simulink model "accBasedController_Simulation"  (R2020a)
settings: Solver=VariableStepAuto  StartTime=0  StopTime=20  FixedStep=0.001  RelTol=1e-3
values from neighbouring files (symbols this model uses):
  A = [0 0 0 1 0 0;      0 0 0 0 1 0;      0 0 0 0 0 1;      -Ka/Jh Ka/Jh 0 0 0 0;     Ka/Je -(Ks + Ka)/Je Ks/Je 0 0 0;      0 Ks/Ja -Ks/Ja 0 0 -Beq/Ja]    [SimulationParam.m]    (also in SimulationParameters.m; abc_ws.mat = [0 0 0 1567.93947765 0 0 0 0 -1685.45584092 221.276595745 0 ; kalmanSS.m = [0 0 0 1 0 0;      0 0 0 0 1 0;      0 0 0 0 0 1;      -Ka/J; kalmanSSHumInput.m = [zeros(1,state_dim);      0 0 0 1 0;      0 0 0 0 1;      Ka)
  A_kf = [0 0 0 0 Ka 0;      0 0 0 0 0 0;      0 0 0 0 1 0;      0 0 0 0 0 1;      0 Ka/Je -(Ks + Ka)/Je Ks/Je 0 0;      0 0 Ks/Ja -Ks/Ja 0 -Beq/Ja]    [SimulationParam.m]    (also in SimulationParameters.m)
  B = [zeros(3,control_dim); 1/Jh 0 0; 0 -1/Je 0; 0 0 N*KI/Ja]    [SimulationParam.m]    (also in SimulationParameters.m; abc_ws.mat = [1 0 0 0 0 0 0 0 -1.12996503145 0 0 0 ... (15 elements, 5x3); kalmanSS.m; kalmanSSHumInput.m = [1 0 0; zeros(2,control_dim); 0 -1/Je 0; 0 0 N*KI/Ja])
  B_kf = [-Ka 0 0; 1 0 0; zeros(2,kf_ctrl_dim); 0 -1/Je 0; 0 0 N*KI/Ja]    [SimulationParam.m]    (also in SimulationParameters.m)
  C = [zeros(sensor_dim,state_dim)]    [SimulationParam.m]    (also in SimulationParameters.m; abc_ws.mat = [-1387.6 0 0 0 0 0 1387.6 0 1 0 0 0 ... (30 elements, 6x5)]; kalmanSS.m; kalmanSSHumInput.m)
  C_kf = [zeros(kf_snr_dim,kf_ste_dim)]    [SimulationParam.m]    (also in SimulationParameters.m)
  CURRENT_MAX = pi    (= 3.14159265359)    [SimulationParam.m]    (also in SimulationParameters.m; abc_ws.mat = 3.14)
  D = zeros(sensor_dim, control_dim)    [SimulationParam.m]    (also in SimulationParameters.m; abc_ws.mat = [0 1 0 0 0 0 0 0 0 0 0 0 ... (18 elements, 6x3)]; kalmanSS.m; kalmanSSHumInput.m = zeros(sensor_dim, control_dim); D(2,1) = 1)
  D_kf = zeros(kf_snr_dim, kf_ctrl_dim); D_kf(2,1) = 1    [SimulationParam.m]    (also in SimulationParameters.m)
  damping_d = 0.001    [SimulationParam.m]    (also in SimulationParameters.m; abc_ws.mat = 0.770835010154; kalmanSSHumInput.m = 0.9)
  dt = 0.001    [SimulationParam.m]    (also in SimulationParameters.m; kalmanSS.m; kalmanSSHumInput.m)
  epos_Ki = 1.190    (= 1.19)    [SimulationParam.m]    (also in SimulationParameters.m; abc_ws.mat; kalmanSSHumInput.m)
  epos_Kp = 11.900    (= 11.9)    [SimulationParam.m]    (also in SimulationParameters.m; abc_ws.mat; kalmanSSHumInput.m)
  Fk = eye(kf_ste_dim) + A_kf*dt + (A_kf*dt)^2/prod(1:2) + (A_kf*dt)^3/prod(1:3) + (A_kf*dt)^4/prod(1:4)    [SimulationParam.m]    (also in SimulationParameters.m; kalmanSS.m = eye(state_dim) + A*dt + (A*dt)^2/prod(1:2) + (A*dt)^3/prod(1; kalmanSSHumInput.m = eye(state_dim) + A*dt + (A*dt)^2/prod(1:2) + (A*dt)^3/prod(1)
  Gk = dt*(eye(kf_ste_dim) + A_kf*dt/prod(1:2) + (A_kf*dt)^2/prod(1:3) + (A_kf*dt)^3/prod(1:4) +         (A_kf*dt)^4/prod(1:5))*B_kf    [SimulationParam.m]    (also in SimulationParameters.m; kalmanSS.m = dt*(eye(state_dim) + A*dt/prod(1:2) + (A*dt)^2/prod(1:3) + (; kalmanSSHumInput.m = dt*(eye(state_dim) + A*dt/prod(1:2) + (A*dt)^2/prod(1:3) + ()
  I_zz = mass_scale*body_mass*(L_leg*r_zz)^2    (= 0.0437446334976)    [SimulationParam.m]    (also in SimulationParameters.m; abc_ws.mat)
  Ja = 0.47    [SimulationParam.m]    (also in SimulationParameters.m; abc_ws.mat; kalmanSS.m; kalmanSSHumInput.m)
  Je = W*Le^2    (= 0.88498313856)    [SimulationParam.m]    (also in SimulationParameters.m; abc_ws.mat; kalmanSS.m; kalmanSSHumInput.m)
  Jh = 0.0437    [SimulationParam.m]    (also in SimulationParameters.m; abc_ws.mat; kalmanSS.m; kalmanSSHumInput.m)
  k_bar = 1 - stiffness_d/Ks    (= 0.993269230769)    [SimulationParam.m]    (also in SimulationParameters.m)
  Ka = Ks/20    (= 5.2)    [SimulationParam.m]    (also in SimulationParameters.m; abc_ws.mat = 1387.6; kalmanSS.m = 1387.6; kalmanSSHumInput.m = 800)
  kf_ste_dim = 6    [SimulationParam.m]    (also in SimulationParameters.m)
  KI = 0.0603    [SimulationParam.m]    (also in SimulationParameters.m; abc_ws.mat; kalmanSS.m; kalmanSSHumInput.m)
  Ks = 104    [SimulationParam.m]    (also in SimulationParameters.m; abc_ws.mat; kalmanSS.m; kalmanSSHumInput.m)
  Le = 0.432    [SimulationParam.m]    (also in SimulationParameters.m; abc_ws.mat; kalmanSS.m; kalmanSSHumInput.m)
  N = 150    [SimulationParam.m]    (also in SimulationParameters.m; abc_ws.mat; kalmanSS.m; kalmanSSHumInput.m)
  p_e_idx = 3    [SimulationParam.m]    (also in SimulationParameters.m)
  p_m_idx = 4    [SimulationParam.m]    (also in SimulationParameters.m)
  Rk = eye(kf_snr_dim)    [SimulationParam.m]    (also in SimulationParameters.m; kalmanSSnoHum.mat = [9.41238823041e-06 0 0 0 0 5.4756e-06 0 0 0 0 2.3530970576e-)
  stiffness_d = 0.7    [SimulationParam.m]    (also in SimulationParameters.m; abc_ws.mat = 14.0803237251; kalmanSSHumInput.m = 3.874)
  stiffness_lower = damping_d*(epos_Ki/epos_Kp - damping_d/(Ja*k_bar) - epos_Kp/Ja)    (= -0.0252212910136)    [SimulationParam.m]    (also in SimulationParameters.m; abc_ws.mat = -20.9019922533; kalmanSSHumInput.m = -24.4873189611)
  Threaded_Ts = 0.001    [SimulationParam.m]    (also in SimulationParameters.m; abc_ws.mat)
  v_e_idx = 5    [SimulationParam.m]    (also in SimulationParameters.m)
  v_h_idx = 2    [SimulationParam.m]    (also in SimulationParameters.m)
  v_m_idx = 6    [SimulationParam.m]    (also in SimulationParameters.m)
  We = W*g    (= 46.5037717323)    [SimulationParam.m]    (also in SimulationParameters.m; abc_ws.mat; kalmanSS.m; kalmanSSHumInput.m)
  zeta = 0.06    [SimulationParam.m]    (also in SimulationParameters.m; abc_ws.mat; kalmanSSHumInput.m = 0.01)
undefined symbols (not defined in the file or in its folder): DiscIntNeverNeededParam, Discrete, Time
libraries: simulink x16, simulink_extras x6, dspstat3 x3, ctrlSharedLib x1
(part 1 of 2)
Description:
  | Collocated Admittance Control study for the acceleration-based SEA Transparency Control
settings Model: OrderedModelArguments=off  Creator=Leonardo Felipe  LastModifiedBy=leona
settings DataIOCC: LimitDataPoints=on  MaxDataPoints=23000  SaveFormat=Array  InspectSignalLogs=on  ReturnWorkspaceOutputs=off
settings SFSimCC: CustomCodeUndefinedFunction=UseInterfaceOnly

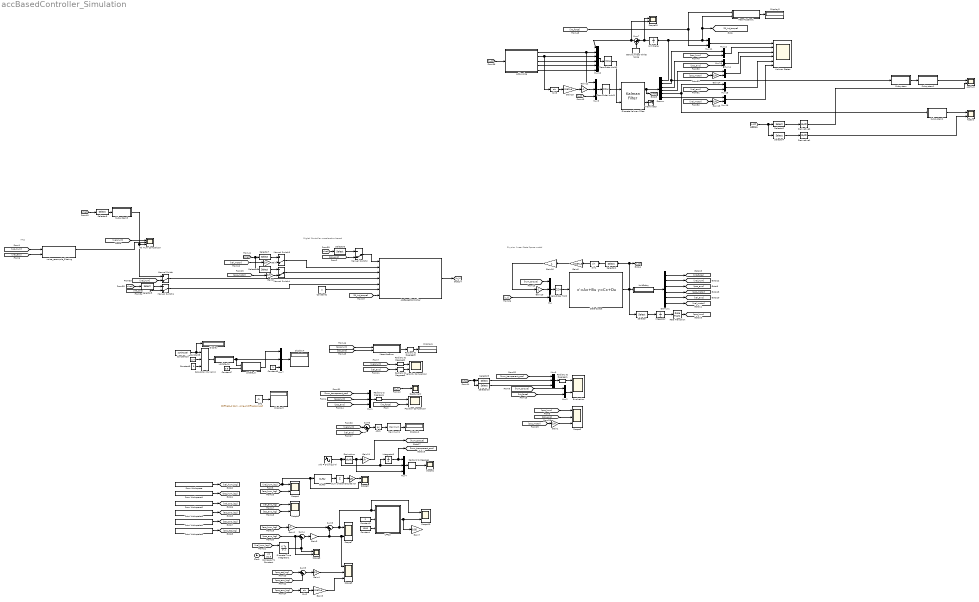
== system accBasedController_Simulation ==
  note: IMUs
  note: Digital Controller: acceleration-based
  note: Physics, linear State Space model
  Abs1 : Abs
  AccBasedController : Subsystem  SystemSampleTime=dt
  AccExo : Scope  NumInputPorts=2
  AccHum : Scope  NumInputPorts=2
  Band-Limited White Noise : simulink/Sources/Band-Limited White Noise  Cov=2*5.476e-6  Ts=dt  seed=[23341]  VectorParams1D=off
  Buffer : Buffer  N=8  OutputFrames=off
  CAC : Constant  Value=[stiffness_d damping_d stiffness_lower]
  Clock : Clock
  Compare To Constant : simulink/Logic and Bit Operations/Compare To Constant  relop=<=  const=32.5  OutDataTypeStr=boolean
  Constant : Constant  Value=1000
  Constant1 : Constant  Value=2
  Constant10 : Constant  Value=sqrt(Ka/Je)
  Constant2 : Constant  Value=2
  Constant5 : Constant
  Constant7 : Constant  Value=0.8
  Constant8 : Constant  Value=2.4
  Constant9 : Constant  Value=0
  DIscrete Kalman Filter : ctrlSharedLib/Kalman Filter  TimeDomain=Discrete-Time  UseCurrentEstimator=on  ModelSource=Individual A, B, C, D matrices  ModelSourceVariable=ss(A_kf, B_kf, C_kf, D_kf)  A=Fk  B=Gk  C=C_kf  D=D_kf  NumberOfStates=1  NumberOfInputs=1  NumberOfOutputs=1  InitialEstimateSource=Dialog  X0=zeros(kf_ste_dim,1)  P0=10  UseK=off  UseGH=off  NumberOfProcessNoiseInputs=1  G=1  TimeInvariantG=on  H=0  TimeInvariantH=on  Q=Qk  TimeInvariantQ=on  R=Rk  TimeInvariantR=on  N=0  TimeInvariantN=on  AddInputPort=on  AddEnablePort=off  OutputEstimatedY=on  OutputP=off  Ts=dt
  Demux : Demux  Outputs=kf_ste_dim
  Demux1 : Demux  Outputs=6
  Derivative : Derivative
  Derivative1 : Derivative
  Derivative2 : Derivative
  DesCurrent : Scope
  Discrete-Time Integrator1 : DiscreteIntegrator  ExternalReset=level  InitialCondition=-0.16  SampleTime=dt  ICPrevOutput=DiscIntNeverNeededParam  ICPrevScaledInput=DiscIntNeverNeededParam
  Display{,2..6} (6 alike) : Display
  Evaluation : Scope  NumInputPorts=2
  From Workspace : FromWorkspace  VariableName=[abc_data.data(:,1) abc_data.data(:,2)]  SampleTime=dt  OutputAfterFinalValue=Holding final value
  From Workspace1 : FromWorkspace  VariableName=[abc_data.data(:,1) abc_data.data(:,4)]  SampleTime=dt  OutputAfterFinalValue=Holding final value
  From Workspace2 : FromWorkspace  VariableName=[abc_data.data(:,1) abc_data.data(:,3)]  SampleTime=dt  OutputAfterFinalValue=Holding final value
  From Workspace3 : FromWorkspace  VariableName=[abc_data.data(:,1) abc_data.data(:,5)]  SampleTime=dt  OutputAfterFinalValue=Holding final value
  From Workspace4 : FromWorkspace  VariableName=[abc_data.data(:,1) abc_data.data(:,7)]  SampleTime=dt  OutputAfterFinalValue=Holding final value
  From Workspace5 : FromWorkspace  VariableName=[abc_data.data(:,1) abc_data.data(:,6)]  SampleTime=dt  OutputAfterFinalValue=Holding final value
  Gain{,1,8,13..14} (5 alike) : Gain  Gain=1/N
  Gain10 : Gain  Gain=-1
  Gain11 : Gain  Gain=Jh
  Gain12 : Gain  Gain=-1
  Gain15 : Gain  Gain=-We*Le
  Gain16 : Gain
  Gain2 : Gain  Gain=Jh
  Gain3 : Gain  Gain=Ks/20
  Gain4 : Gain  Gain=Ks
  Gain5 : Gain  Gain=-We*Le
  Gain6 : Gain  Gain=-We*Le
  Gain7 : Gain  Gain=0.05
  Gain9 : Gain  Gain=1/8
  Integrator : Integrator
  Integrator3 : Integrator
  Kalman States : Scope  NumInputPorts=6
  LPF2p : Subsystem
  Manual Switch{,1..4} (5 alike) : ManualSwitch  CurrentSetting=0
  Maximum1 : dspstat3/Maximum  operation=maximum  fcn=Running  indexBase=One  operateOver=Each column  Dimension=1  InputProcessing=Columns as channels (frame based)  reset=None  roiEnable=off  roiType=Rectangles  roiPortion=Entire ROI  roiOutput=Individual statistics for each ROI  roiFlag=off  roundingMode=Floor  overflowMode=off  accumDataTypeStr=Inherit: Same as product output  accumLastDataTypeStr=Inherit: Same as product output
  MeanAbsError : Subsystem
  MeanAbsError1 : Subsystem
  Mux{,1,3..4,7,9} (6 alike) : Mux  Inputs=3
  Mux10 : Mux  Inputs=kf_snr_dim
  Mux{2,11..16} (7 alike) : Mux  Inputs=2
  Position Comparison : Scope  NumInputPorts=2
  Radians to Degrees{,1..5} (6 alike) : simulink_extras/Transformations/Radians to Degrees
  Rate Transition : RateTransition  OutPortSampleTime=dt
  Saturation Dynamic : simulink/Discontinuities/Saturation Dynamic  OutMin=[]  OutMax=[]  OutDataTypeStr=Inherit: Same as second input  OutDataType=fixdt(1, 16)  OutScaling=2^-10  DoSatur=off
  Scope1 : Scope
  Scope{3..5,7..8,10,18} (7 alike) : Scope  NumInputPorts=2
  Scope6 : Scope  NumInputPorts=3
  Scope9 : Scope  NumInputPorts=3
  Selector : Selector  InputPortWidth=sensor_dim  IndexOptions=Index vector (dialog)  Indices=[v_h_idx]  OutputSizes=1
  Selector1 : Selector  InputPortWidth=sensor_dim  IndexOptions=Index vector (dialog)  Indices=[p_e_idx]  OutputSizes=1
  Selector10 : Selector  InputPortWidth=kf_ste_dim  IndexOptions=Index vector (dialog)  Indices=[3]  OutputSizes=1
  Selector2 : Selector  InputPortWidth=sensor_dim  IndexOptions=Index vector (dialog)  Indices=[v_h_idx]  OutputSizes=1
  Selector3 : Selector  InputPortWidth=kf_ste_dim  IndexOptions=Index vector (dialog)  Indices=[2]  OutputSizes=1
  Selector4 : Selector  InputPortWidth=sensor_dim  IndexOptions=Index vector (dialog)  Indices=[v_e_idx]  OutputSizes=1
  Selector5 : Selector  InputPortWidth=kf_ste_dim  IndexOptions=Index vector (dialog)  Indices=[5]  OutputSizes=1
  Selector6 : Selector  InputPortWidth=kf_ste_dim  IndexOptions=Index vector (dialog)  Indices=[3]  OutputSizes=1
  Selector7 : Selector  InputPortWidth=kf_ste_dim  IndexOptions=Index vector (dialog)  Indices=[6]  OutputSizes=1
  Selector8 : Selector  InputPortWidth=kf_ste_dim  IndexOptions=Index vector (dialog)  Indices=[4]  OutputSizes=1
  Selector9 : Selector  InputPortWidth=kf_ste_dim  IndexOptions=Index vector (dialog)  Indices=[2]  OutputSizes=1
  Sin1 : Trigonometry
  Sin2 : Trigonometry
  Sin3 : Trigonometry
  State-Space : StateSpace  A=A  B=B  C=C  D=D  InitialCondition=0  ContinuousStateAttributes={'x_h','x_e','x_a','dx_h','dx_e','dx_a'}
  Subsystem : Subsystem
  Subsystem1 : Subsystem
  Subsystem2 : Subsystem
  Subsystem3 : Subsystem
  Sum of Elements : Sum  Inputs=+
  Sum{3..6} (4 alike) : Sum  Inputs=|+-
  Sum7 : Sum  Inputs=|++
  Terminator : Terminator
  Unit Delay : UnitDelay  SampleTime=-1  HasFrameUpgradeWarning=on
  UnitDelay : Subsystem  TreatAsAtomicUnit=on  SystemSampleTime=dt
  Vel Hum Comparison : Scope  NumInputPorts=3
  Velocity Comparison : Scope  NumInputPorts=2
  Zero-Order Hold : ZeroOrderHold  SampleTime=Threaded_Ts
  Zero-Order Hold1 : ZeroOrderHold  SampleTime=dt
  Zero-Order Hold2 : ZeroOrderHold  SampleTime=dt
  add_noise : Subsystem
  noise_resample_filtering : Subsystem
  update_Ki : Subsystem
  update_Kp : Subsystem
  w(t) = 3*sin(2pi*t) : Sin  Amplitude=3  Frequency=4*pi  SampleTime=0
  wires:
  Zero-Order Hold/1 -> State-Space/1  "u"
  State-Space/1 -> Selector/1, UnitDelay/1(In1), [y_ss], Selector1/1  "z"
  Mux/1 -> Zero-Order Hold/1
  UnitDelay/1(y) -> Demux1/1  "y"
  [vel_hum] -> Radians to Degrees2/1
  [vel_exo] -> Radians to Degrees3/1
  [pos_hum] -> Scope6/1  "pos_hum"
  [pos_exo] -> Scope6/2  "pos_exo"
  Constant2/1 -> AccBasedController/6(control_type)  "controller"
  [vel_motor] -> Gain/1
  Sin1/1 -> Gain6/1
  Demux1/3 -> [pos_exo]
  AccBasedController/1(DesCurrent) -> [u_k]  "I"
  [pos_motor] -> Gain1/1
  Radians to Degrees2/1 -> Velocity Comparison/1
  Radians to Degrees3/1 -> Velocity Comparison/2
  [u_k] -> DesCurrent/1  "control"
  Gain10/1 -> Mux/2
  [vel_hum] -> Vel Hum Comparison/1
  Demux1/2 -> [vel_hum]
  Demux1/1 -> [int_force]
  Demux1/4 -> [pos_motor]
  Demux1/5 -> [vel_exo]
  Demux1/6 -> [vel_motor]
  Mux1/1 -> Radians to Degrees4/1
  Radians to Degrees4/1 -> Position Comparison/1
  [int_force] -> Position Comparison/2  "t_i"
  [hum_torque] -> Mux/1
  Gain1/1 -> Scope6/3  "pos_act"
  From Workspace/1 -> [vel_hum_log]
  From Workspace1/1 -> [acc_hum_log]
  From Workspace3/1 -> [acc_exo_log]
  From Workspace2/1 -> [vel_exo_log]
  [acc_hum_log] -> Scope4/2
  [vel_hum_log] -> Scope3/2, Buffer/1, Scope4/1
  [acc_exo_log] -> Scope5/2
  [vel_exo_log] -> Scope5/1
  [acc_hum_log] -> Gain2/1
  Gain2/1 -> Sum3/1
  Sum4/1 -> Gain3/1
  Gain3/1 -> Sum3/2, Scope9/1, Scope7/2  "F_i"
  From Workspace4/1 -> [pos_exo_log]
  [pos_exo_log] -> Scope8/2, Sum4/1
  [vel_hum_log] -> Discrete-Time Integrator1/1
  Discrete-Time Integrator1/1 -> Sum4/2, Scope8/1  "pos_hum"
  Sum3/1 -> Scope10/1, LPF2p/1(sample), Scope7/1  "F_h"
  Clock/1 -> Compare To Constant/1
  From Workspace5/1 -> [pos_act_log]
  Sum5/1 -> Gain4/1
  [pos_act_log] -> Sum5/1
  [pos_exo_log] -> Sum5/2
  Gain4/1 -> Scope9/2  "F_s"
  Gain5/1 -> Scope9/3  "F_W"
  Sin2/1 -> Gain5/1
  [pos_exo_log] -> Sin2/1
  Constant/1 -> LPF2p/3(sample_freq)
  Constant1/1 -> LPF2p/2(cutoff_freq)
  LPF2p/1(output) -> Scope10/2, Gain7/1
  [vel_hum] -> Sum6/1
  [vel_exo] -> Sum6/2
  Abs1/1 -> Maximum1/1
  Maximum1/1 -> Display2/1
  Sum6/1 -> Abs1/1
  [pos_motor] -> Gain8/1
  CAC/1 -> Display3/1
  Selector/1 -> Integrator/1
  Integrator/1 -> Rate Transition/1
  Rate Transition/1 -> [pos_hum]
  Selector1/1 -> Sin1/1
  [u_k] -> Mux/3
  [vel_hum] -> noise_resample_filtering/1(vel_hum)
  [vel_exo] -> noise_resample_filtering/2(vel_exo)
  Mux3/1 -> Radians to Degrees1/1
  Selector10/1 -> Mux3/3  "pos_e"
  Selector9/1 -> Mux3/2  "pos_h"
  [hum_torque] -> Mux2/1  "T_h"
  [int_force] -> Mux2/2  "T_i"
  Mux2/1 -> Evaluation/2
  Radians to Degrees1/1 -> Evaluation/1
  [pos_exo] -> Mux1/3  "pos_e"
  [pos_hum] -> Mux1/2  "pos_h"
  [hum_transparent_pos] -> Mux1/1  "pos_h_trans"
  w(t) = 3*sin(2pi*t)/1 -> Integrator3/1, Mux4/2, Derivative/1  "v"
  Derivative/1 -> Mux4/3, Gain11/1  "a"
  Integrator3/1 -> [hum_transparent_pos], Mux4/1  "p"
  Mux4/1 -> Radians to Degrees/1
  Gain11/1 -> [hum_torque]  "T"
  Radians to Degrees/1 -> Scope1/1
  Constant5/1 -> Mux7/3
  Mux7/1 -> Display4/1  "Abc"
  update_Kp/1(Kp_acc) -> Mux7/2, update_Ki/1(Kp_acc)
  update_Ki/1(Ki_acc) -> Mux7/1
  Constant7/1 -> update_Ki/2(zeta)
  Constant9/1 -> Saturation Dynamic/3
  Constant8/1 -> Saturation Dynamic/2
  Saturation Dynamic/1 -> update_Kp/1(w_n)
  Constant10/1 -> Display/1, Saturation Dynamic/1
  [hum_transparent_pos] -> Mux3/1  "pos_h_trans"
  Buffer/1 -> Sum of Elements/1
  Sum of Elements/1 -> Gain9/1
  Gain9/1 -> Scope3/1
  add_noise/1(vel_hum_corr) -> Mux10/2, Mux9/1
  Gain12/1 -> Mux9/2
  Mux9/1 -> Zero-Order Hold1/1
  Zero-Order Hold1/1 -> DIscrete Kalman Filter/1  "u"
  [u_k] -> Mux9/3
  DIscrete Kalman Filter/1 -> [xhat], Demux/1
  Mux10/1 -> Zero-Order Hold2/1
  add_noise/4(vel_exo_corr) -> Mux10/5
  Zero-Order Hold2/1 -> DIscrete Kalman Filter/2  "u"
  [int_force] -> MeanAbsError1/1(ref), Mux11/2
  [pos_exo] -> Mux13/2
  Demux/3 -> Mux13/1  "x_e"
  Demux/1 -> MeanAbsError1/2(state), [kf_int_torque], Mux11/1, Unit Delay/1  "t_i"
  Demux/2 -> Mux12/1, Subsystem/1(x)  "x_h"
  [pos_hum] -> Mux12/2
  Demux/4 -> Mux14/1  "x_a"
  [pos_motor] -> Gain14/1
  Gain14/1 -> Mux14/2
  [vel_motor] -> Gain13/1
  [vel_exo] -> Mux15/2
  Demux/5 -> Mux15/1, Subsystem2/1(x)  "dot_x_e"
  Band-Limited White Noise/1 -> Sum7/2
  Sum7/1 -> Scope18/2, Mux10/1
  add_noise/2(pos_exo_corr) -> Sin3/1, Mux10/3
  add_noise/3(pos_motor_corr) -> Mux10/4
  add_noise/5(vel_motor_corr) -> Mux10/6
  Unit Delay/1 -> Scope18/1, Sum7/1
  Sin3/1 -> Gain15/1
  Gain15/1 -> Gain12/1
  Mux11/1 -> Kalman States/1  "t_i"
  Mux12/1 -> Kalman States/2  "x_h"
  Mux13/1 -> Kalman States/3  "x_e"
  Mux14/1 -> Kalman States/4  "x_a"
  Gain13/1 -> Mux16/2
  Demux/6 -> Mux16/1  "dot_x_a"
  Mux15/1 -> Kalman States/5  "dot_x_e"
  Mux16/1 -> Kalman States/6  "dot_x_a"
  [kf_int_torque] -> AccBasedController/7(int_torque_est)
  DIscrete Kalman Filter/2 -> Terminator/1
  Selector2/1 -> Derivative2/1
  Subsystem/1(dot_x) -> Subsystem1/1(x)
  Selector4/1 -> Derivative1/1
  [pos_hum] -> MeanAbsError/1(ref)  "pos_h"
  [pos_exo] -> MeanAbsError/2(state)  "pos_e"
  MeanAbsError/1(Error) -> Radians to Degrees5/1
  MeanAbsError1/1(Error) -> Display5/1
  Subsystem1/1(dot_x) -> AccHum/1
  Derivative2/1 -> AccHum/2
  Subsystem2/1(dot_x) -> AccExo/1
  Derivative1/1 -> AccExo/2
  Gain6/1 -> Gain16/1
  Radians to Degrees5/1 -> Display6/1
  noise_resample_filtering/1(ve_hum_filt) -> Vel Hum Comparison/2
  [y_ss] -> Selector4/1, Selector2/1
  [y_ss] -> add_noise/1(y)
  Subsystem3/1(dot_x) -> Manual Switch/1, Vel Hum Comparison/3
  Manual Switch/1 -> AccBasedController/4(vel_hum)
  Selector5/1 -> Manual Switch1/1
  Manual Switch1/1 -> AccBasedController/5(vel_exo)
  Gain16/1 -> Gain10/1
  [xhat] -> Selector3/1
  Selector3/1 -> Subsystem3/1(x)
  [xhat] -> Selector5/1
  [xhat] -> Selector6/1
  Manual Switch2/1 -> AccBasedController/1(pos_exo)
  [pos_exo] -> Manual Switch2/2
  Selector6/1 -> Manual Switch2/1
  Gain/1 -> Manual Switch3/2
  Selector7/1 -> Manual Switch3/1
  Manual Switch3/1 -> AccBasedController/2(vel_actuator)
  Selector8/1 -> Manual Switch4/1
  [xhat] -> Selector8/1, Selector7/1
  Gain8/1 -> Manual Switch4/2
  Manual Switch4/1 -> AccBasedController/3(pos_act)
  [xhat] -> Selector10/1, Selector9/1
  [vel_exo] -> Manual Switch1/2
  [vel_hum] -> Manual Switch/2

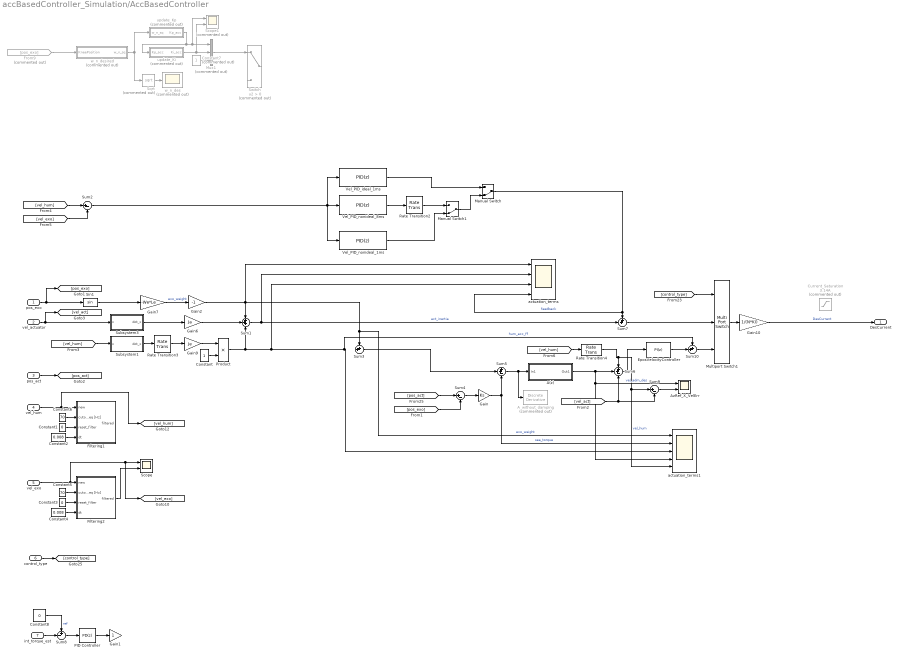
== system accBasedController_Simulation/AccBasedController ==
  pos_exo : Inport
  vel_actuator : Inport  Port=2
  pos_act : Inport  Port=3
  vel_hum : Inport  Port=4
  vel_exo : Inport  Port=5
  control_type : Inport  Port=6
  int_torque_est : Inport  Port=7
  A(z) : Subsystem
  A_without_damping : simulink/Discrete/Discrete Derivative  Commented=on  gainval=k_bar/stiffness_d  ICPrevScaledInput=0.0  OutMin=[]  OutMax=[]  OutDataType=fixdt(1, 16)  OutScaling=2^-10  DoSatur=off
  AzRef_X_VelErr : Scope  NumInputPorts=2
  Constant : Constant
  Constant1 : Constant  Value=0
  Constant2 : Constant  Value=0.008
  Constant3 : Constant  Value=0
  Constant4 : Constant  Value=0.008
  Constant5 : Constant  Value=70
  Constant6 : Constant  Value=70
  Constant7 : Constant  Commented=on
  Constant8 : Constant  Value=0
  Current_Saturation 3.14A : Saturate  Commented=on  UpperLimit=CURRENT_MAX  LowerLimit=-CURRENT_MAX
  EposVelocityController : simulink/Continuous/PID Controller  Controller=PI  Form=Parallel  TimeDomain=Discrete-time  UseExternalTs=off  SampleTime=dt  IntegratorMethod=Forward Euler  FilterMethod=Forward Euler  ControllerParametersSource=internal  P=epos_Kp  I=epos_Ki  D=279.805559989798  UseFilter=off  N=100  TunerSelectOption=Transfer Function Based (PID Tuner App)  InitialConditionSource=internal  InitialConditionForIntegrator=0  InitialConditionForFilter=0  DifferentiatorICPrevScaledInput=0  ExternalReset=none  TrackingMode=off  Kt=1  LimitOutput=off  UpperSaturationLimit=inf  LowerSaturationLimit=-inf  LinearizeAsGain=on  AntiWindupMode=none  Kb=1  POutMin=[]  POutMax=[]  IOutMin=[]  IOutMax=[]  DOutMin=[]  DOutMax=[]  NOutMin=[]  NOutMax=[]  SumOutMin=[]  SumOutMax=[]  SaturationOutMin=[]  SaturationOutMax=[]  PParamMin=[]  PParamMax=[]  IParamMin=[]  IParamMax=[]  DParamMin=[]  DParamMax=[]  NParamMin=[]  NParamMax=[]  KbParamMin=[]  KbParamMax=[]  KtParamMin=[]  KtParamMax=[]  KbOutMin=[]  KbOutMax=[]  KtOutMin=[]  KtOutMax=[]  IntegratorOutMin=[]  IntegratorOutMax=[]  FilterOutMin=[]  FilterOutMax=[]  SumI1OutMin=[]  SumI1OutMax=[]  SumI2OutMin=[]  SumI2OutMax=[]  SumI3OutMin=[]  SumI3OutMax=[]  SumI4OutMin=[]  SumI4OutMax=[]  SumDOutMin=[]  SumDOutMax=[]  DifferentiatorOutMin=[]  DifferentiatorOutMax=[]  FilterDiffOutCoefMin=[]  FilterDiffOutCoefMax=[]  ReciprocalOutMin=[]  ReciprocalOutMax=[]  SumDenOutMin=[]  SumDenOutMax=[]  SumNumOutMin=[]  SumNumOutMax=[]  DivideOutMin=[]  DivideOutMax=[]  UdiffTsProdOutMin=[]  UdiffTsProdOutMax=[]  NTsProdOutMin=[]  NTsProdOutMax=[]  UintegralTsProdOutMin=[]  UintegralTsProdOutMax=[]  UngainTsProdOutMin=[]  UngainTsProdOutMax=[]  IntegratorContinuousStateAttributes=''  IntegratorStateMustResolveToSignalObject=off  IntegratorRTWStateStorageClass=Auto  FilterContinuousStateAttributes=''  FilterStateMustResolveToSignalObject=off  FilterRTWStateStorageClass=Auto  ParallelPVariant=InternalParameters  IdealPVariant=Disabled  IVariant=InternalParameters  DVariant=Disabled  IntegratorVariant=Discrete  SatVariant=Disabled  AWVariant=Passthrough  PCopyVariant=Disabled  TRVariant=Disabled  FdbkBlocksVariant=Forward  IdealPFdbkVariant=Disabled  SatFdbkVariant=Disabled  DerivativeFilterVariant=Disabled  NVariant=Disabled  NCopyVariant=Disabled_SignalSpec  FilterICVariant=Disabled  IntegratorICVariant=InternalICs  ExternalResetVariant=Disabled  TRSumVariant=Passthrough  SumFdbkVariant=Disabled  SumVariant=Sum_PI  TsampFilterVariant=InternalTs  TsampNgainVariant=Passthrough  TsampIntegralVariant=Passthrough
  Filtering1 : Subsystem
  Filtering2 : Subsystem
  From9 : From  Commented=on  GotoTag=pos_exo
  Gain : Gain  Gain=Ks
  Gain1 : Gain
  Gain10 : Gain  Gain=1/(N*KI)
  Gain2 : Gain  Gain=-1
  Gain6 : Gain  Gain=Ja
  Gain7 : Gain  Gain=-We*Le
  Gain9 : Gain  Gain=Je
  Manual Switch : ManualSwitch  CurrentSetting=0
  Manual Switch1 : ManualSwitch  CurrentSetting=0
  Multiport Switch1 : MultiPortSwitch  Inputs=2
  Mux1 : Mux  Commented=on  Inputs=3
  PID Controller : simulink/Continuous/PID Controller  Controller=PD  Form=Parallel  TimeDomain=Discrete-time  UseExternalTs=off  SampleTime=dt  IntegratorMethod=Forward Euler  FilterMethod=Forward Euler  ControllerParametersSource=internal  P=23  I=1  D=1.6  UseFilter=on  N=100  TunerSelectOption=Transfer Function Based (PID Tuner App)  InitialConditionSource=internal  InitialConditionForIntegrator=0  InitialConditionForFilter=0  DifferentiatorICPrevScaledInput=0  ExternalReset=none  TrackingMode=off  Kt=1  LimitOutput=off  UpperSaturationLimit=inf  LowerSaturationLimit=-inf  LinearizeAsGain=on  AntiWindupMode=none  Kb=1  POutMin=[]  POutMax=[]  IOutMin=[]  IOutMax=[]  DOutMin=[]  DOutMax=[]  NOutMin=[]  NOutMax=[]  SumOutMin=[]  SumOutMax=[]  SaturationOutMin=[]  SaturationOutMax=[]  PParamMin=[]  PParamMax=[]  IParamMin=[]  IParamMax=[]  DParamMin=[]  DParamMax=[]  NParamMin=[]  NParamMax=[]  KbParamMin=[]  KbParamMax=[]  KtParamMin=[]  KtParamMax=[]  KbOutMin=[]  KbOutMax=[]  KtOutMin=[]  KtOutMax=[]  IntegratorOutMin=[]  IntegratorOutMax=[]  FilterOutMin=[]  FilterOutMax=[]  SumI1OutMin=[]  SumI1OutMax=[]  SumI2OutMin=[]  SumI2OutMax=[]  SumI3OutMin=[]  SumI3OutMax=[]  SumI4OutMin=[]  SumI4OutMax=[]  SumDOutMin=[]  SumDOutMax=[]  DifferentiatorOutMin=[]  DifferentiatorOutMax=[]  FilterDiffOutCoefMin=[]  FilterDiffOutCoefMax=[]  ReciprocalOutMin=[]  ReciprocalOutMax=[]  SumDenOutMin=[]  SumDenOutMax=[]  SumNumOutMin=[]  SumNumOutMax=[]  DivideOutMin=[]  DivideOutMax=[]  UdiffTsProdOutMin=[]  UdiffTsProdOutMax=[]  NTsProdOutMin=[]  NTsProdOutMax=[]  UintegralTsProdOutMin=[]  UintegralTsProdOutMax=[]  UngainTsProdOutMin=[]  UngainTsProdOutMax=[]  IntegratorContinuousStateAttributes=''  IntegratorStateMustResolveToSignalObject=off  IntegratorRTWStateStorageClass=Auto  FilterContinuousStateAttributes=''  FilterStateMustResolveToSignalObject=off  FilterRTWStateStorageClass=Auto  ParallelPVariant=InternalParameters  IdealPVariant=Disabled  IVariant=Disabled  DVariant=InternalParameters  IntegratorVariant=Disabled  SatVariant=Disabled  AWVariant=Disabled  PCopyVariant=Disabled  TRVariant=Disabled  FdbkBlocksVariant=Forward  IdealPFdbkVariant=Disabled  SatFdbkVariant=Disabled  DerivativeFilterVariant=ForwardEulerFilter  NVariant=InternalParameters  NCopyVariant=Disabled  FilterICVariant=InternalICsFilter  IntegratorICVariant=Disabled  ExternalResetVariant=Disabled  TRSumVariant=Passthrough  SumFdbkVariant=Disabled  SumVariant=Sum_PD  TsampFilterVariant=InternalTs  TsampNgainVariant=Passthrough  TsampIntegralVariant=Disabled_SignalSpec
  Product : Product
  Rate Transition2 : RateTransition  OutPortSampleTime=0.001
  Rate Transition3 : RateTransition  OutPortSampleTime=0.001
  Rate Transition4 : RateTransition  OutPortSampleTime=0.001
  Scope : Scope  NumInputPorts=2
  Scope1 : Scope  Commented=on  NumInputPorts=2
  Sin1 : Trigonometry
  Sqrt : Sqrt  Commented=on  SaturateOnIntegerOverflow=on
  Subsystem1 : Subsystem
  Subsystem3 : Subsystem
  Sum1 : Sum  Inputs=+++
  Sum10 : Sum  Inputs=++|
  Sum2 : Sum  Inputs=|+-
  Sum3 : Sum  Inputs=++|
  Sum4 : Sum  Inputs=|+-
  Sum5 : Sum  Inputs=++-
  Sum6 : Sum  Inputs=++-
  Sum7 : Sum  Inputs=++|
  Sum8 : Sum  Inputs=+-|
  Sum9 : Sum  Inputs=|+-
  Switch : Switch  Commented=on  Criteria=u2 > Threshold
  Vel_PID_ideal_1ms : simulink/Continuous/PID Controller  Controller=PID  Form=Parallel  TimeDomain=Discrete-time  UseExternalTs=off  SampleTime=dt  IntegratorMethod=Forward Euler  FilterMethod=Forward Euler  ControllerParametersSource=internal  P=410  I=330  D=0.15  UseFilter=off  N=100  TunerSelectOption=Transfer Function Based (PID Tuner App)  InitialConditionSource=internal  InitialConditionForIntegrator=0  InitialConditionForFilter=0  DifferentiatorICPrevScaledInput=0  ExternalReset=none  TrackingMode=off  Kt=1  LimitOutput=off  UpperSaturationLimit=inf  LowerSaturationLimit=-inf  LinearizeAsGain=on  AntiWindupMode=none  Kb=1  POutMin=[]  POutMax=[]  IOutMin=[]  IOutMax=[]  DOutMin=[]  DOutMax=[]  NOutMin=[]  NOutMax=[]  SumOutMin=[]  SumOutMax=[]  SaturationOutMin=[]  SaturationOutMax=[]  PParamMin=[]  PParamMax=[]  IParamMin=[]  IParamMax=[]  DParamMin=[]  DParamMax=[]  NParamMin=[]  NParamMax=[]  KbParamMin=[]  KbParamMax=[]  KtParamMin=[]  KtParamMax=[]  KbOutMin=[]  KbOutMax=[]  KtOutMin=[]  KtOutMax=[]  IntegratorOutMin=[]  IntegratorOutMax=[]  FilterOutMin=[]  FilterOutMax=[]  SumI1OutMin=[]  SumI1OutMax=[]  SumI2OutMin=[]  SumI2OutMax=[]  SumI3OutMin=[]  SumI3OutMax=[]  SumI4OutMin=[]  SumI4OutMax=[]  SumDOutMin=[]  SumDOutMax=[]  DifferentiatorOutMin=[]  DifferentiatorOutMax=[]  FilterDiffOutCoefMin=[]  FilterDiffOutCoefMax=[]  ReciprocalOutMin=[]  ReciprocalOutMax=[]  SumDenOutMin=[]  SumDenOutMax=[]  SumNumOutMin=[]  SumNumOutMax=[]  DivideOutMin=[]  DivideOutMax=[]  UdiffTsProdOutMin=[]  UdiffTsProdOutMax=[]  NTsProdOutMin=[]  NTsProdOutMax=[]  UintegralTsProdOutMin=[]  UintegralTsProdOutMax=[]  UngainTsProdOutMin=[]  UngainTsProdOutMax=[]  IntegratorContinuousStateAttributes=''  IntegratorStateMustResolveToSignalObject=off  IntegratorRTWStateStorageClass=Auto  FilterContinuousStateAttributes=''  FilterStateMustResolveToSignalObject=off  FilterRTWStateStorageClass=Auto  ParallelPVariant=InternalParameters  IdealPVariant=Disabled  IVariant=InternalParameters  DVariant=InternalParameters  IntegratorVariant=Discrete  SatVariant=Disabled  AWVariant=Passthrough  PCopyVariant=Disabled  TRVariant=Disabled  FdbkBlocksVariant=Forward  IdealPFdbkVariant=Disabled  SatFdbkVariant=Disabled  DerivativeFilterVariant=Differentiator  NVariant=Passthrough  NCopyVariant=Disabled_SignalSpec  FilterICVariant=InternalICsDifferentiator  IntegratorICVariant=InternalICs  ExternalResetVariant=Disabled  TRSumVariant=Passthrough  SumFdbkVariant=Disabled  SumVariant=Sum_PID  TsampFilterVariant=InternalTs  TsampNgainVariant=Passthrough  TsampIntegralVariant=Passthrough
  Vel_PID_nonideal_1ms : simulink/Continuous/PID Controller  Controller=PID  Form=Parallel  TimeDomain=Discrete-time  UseExternalTs=off  SampleTime=dt  IntegratorMethod=Forward Euler  FilterMethod=Forward Euler  ControllerParametersSource=internal  P=346.80  I=0  D=4.92  UseFilter=off  N=100  TunerSelectOption=Transfer Function Based (PID Tuner App)  InitialConditionSource=internal  InitialConditionForIntegrator=0  InitialConditionForFilter=0  DifferentiatorICPrevScaledInput=0  ExternalReset=none  TrackingMode=off  Kt=1  LimitOutput=off  UpperSaturationLimit=inf  LowerSaturationLimit=-inf  LinearizeAsGain=on  AntiWindupMode=none  Kb=1  POutMin=[]  POutMax=[]  IOutMin=[]  IOutMax=[]  DOutMin=[]  DOutMax=[]  NOutMin=[]  NOutMax=[]  SumOutMin=[]  SumOutMax=[]  SaturationOutMin=[]  SaturationOutMax=[]  PParamMin=[]  PParamMax=[]  IParamMin=[]  IParamMax=[]  DParamMin=[]  DParamMax=[]  NParamMin=[]  NParamMax=[]  KbParamMin=[]  KbParamMax=[]  KtParamMin=[]  KtParamMax=[]  KbOutMin=[]  KbOutMax=[]  KtOutMin=[]  KtOutMax=[]  IntegratorOutMin=[]  IntegratorOutMax=[]  FilterOutMin=[]  FilterOutMax=[]  SumI1OutMin=[]  SumI1OutMax=[]  SumI2OutMin=[]  SumI2OutMax=[]  SumI3OutMin=[]  SumI3OutMax=[]  SumI4OutMin=[]  SumI4OutMax=[]  SumDOutMin=[]  SumDOutMax=[]  DifferentiatorOutMin=[]  DifferentiatorOutMax=[]  FilterDiffOutCoefMin=[]  FilterDiffOutCoefMax=[]  ReciprocalOutMin=[]  ReciprocalOutMax=[]  SumDenOutMin=[]  SumDenOutMax=[]  SumNumOutMin=[]  SumNumOutMax=[]  DivideOutMin=[]  DivideOutMax=[]  UdiffTsProdOutMin=[]  UdiffTsProdOutMax=[]  NTsProdOutMin=[]  NTsProdOutMax=[]  UintegralTsProdOutMin=[]  UintegralTsProdOutMax=[]  UngainTsProdOutMin=[]  UngainTsProdOutMax=[]  IntegratorContinuousStateAttributes=''  IntegratorStateMustResolveToSignalObject=off  IntegratorRTWStateStorageClass=Auto  FilterContinuousStateAttributes=''  FilterStateMustResolveToSignalObject=off  FilterRTWStateStorageClass=Auto  ParallelPVariant=InternalParameters  IdealPVariant=Disabled  IVariant=InternalParameters  DVariant=InternalParameters  IntegratorVariant=Discrete  SatVariant=Disabled  AWVariant=Passthrough  PCopyVariant=Disabled  TRVariant=Disabled  FdbkBlocksVariant=Forward  IdealPFdbkVariant=Disabled  SatFdbkVariant=Disabled  DerivativeFilterVariant=Differentiator  NVariant=Passthrough  NCopyVariant=Disabled_SignalSpec  FilterICVariant=InternalICsDifferentiator  IntegratorICVariant=InternalICs  ExternalResetVariant=Disabled  TRSumVariant=Passthrough  SumFdbkVariant=Disabled  SumVariant=Sum_PID  TsampFilterVariant=InternalTs  TsampNgainVariant=Passthrough  TsampIntegralVariant=Passthrough
  Vel_PID_nonideal_8ms : simulink/Continuous/PID Controller  Controller=PID  Form=Parallel  TimeDomain=Discrete-time  UseExternalTs=off  SampleTime=8*dt  IntegratorMethod=Forward Euler  FilterMethod=Forward Euler  ControllerParametersSource=internal  P=346.80  I=18  D=4.92  UseFilter=off  N=100  TunerSelectOption=Transfer Function Based (PID Tuner App)  InitialConditionSource=internal  InitialConditionForIntegrator=0  InitialConditionForFilter=0  DifferentiatorICPrevScaledInput=0  ExternalReset=none  TrackingMode=off  Kt=1  LimitOutput=off  UpperSaturationLimit=inf  LowerSaturationLimit=-inf  LinearizeAsGain=on  AntiWindupMode=none  Kb=1  POutMin=[]  POutMax=[]  IOutMin=[]  IOutMax=[]  DOutMin=[]  DOutMax=[]  NOutMin=[]  NOutMax=[]  SumOutMin=[]  SumOutMax=[]  SaturationOutMin=[]  SaturationOutMax=[]  PParamMin=[]  PParamMax=[]  IParamMin=[]  IParamMax=[]  DParamMin=[]  DParamMax=[]  NParamMin=[]  NParamMax=[]  KbParamMin=[]  KbParamMax=[]  KtParamMin=[]  KtParamMax=[]  KbOutMin=[]  KbOutMax=[]  KtOutMin=[]  KtOutMax=[]  IntegratorOutMin=[]  IntegratorOutMax=[]  FilterOutMin=[]  FilterOutMax=[]  SumI1OutMin=[]  SumI1OutMax=[]  SumI2OutMin=[]  SumI2OutMax=[]  SumI3OutMin=[]  SumI3OutMax=[]  SumI4OutMin=[]  SumI4OutMax=[]  SumDOutMin=[]  SumDOutMax=[]  DifferentiatorOutMin=[]  DifferentiatorOutMax=[]  FilterDiffOutCoefMin=[]  FilterDiffOutCoefMax=[]  ReciprocalOutMin=[]  ReciprocalOutMax=[]  SumDenOutMin=[]  SumDenOutMax=[]  SumNumOutMin=[]  SumNumOutMax=[]  DivideOutMin=[]  DivideOutMax=[]  UdiffTsProdOutMin=[]  UdiffTsProdOutMax=[]  NTsProdOutMin=[]  NTsProdOutMax=[]  UintegralTsProdOutMin=[]  UintegralTsProdOutMax=[]  UngainTsProdOutMin=[]  UngainTsProdOutMax=[]  IntegratorContinuousStateAttributes=''  IntegratorStateMustResolveToSignalObject=off  IntegratorRTWStateStorageClass=Auto  FilterContinuousStateAttributes=''  FilterStateMustResolveToSignalObject=off  FilterRTWStateStorageClass=Auto  ParallelPVariant=InternalParameters  IdealPVariant=Disabled  IVariant=InternalParameters  DVariant=InternalParameters  IntegratorVariant=Discrete  SatVariant=Disabled  AWVariant=Passthrough  PCopyVariant=Disabled  TRVariant=Disabled  FdbkBlocksVariant=Forward  IdealPFdbkVariant=Disabled  SatFdbkVariant=Disabled  DerivativeFilterVariant=Differentiator  NVariant=Passthrough  NCopyVariant=Disabled_SignalSpec  FilterICVariant=InternalICsDifferentiator  IntegratorICVariant=InternalICs  ExternalResetVariant=Disabled  TRSumVariant=Passthrough  SumFdbkVariant=Disabled  SumVariant=Sum_PID  TsampFilterVariant=InternalTs  TsampNgainVariant=Passthrough  TsampIntegralVariant=Passthrough
  actuation_terms : Scope  NumInputPorts=4
  actuation_terms1 : Scope  NumInputPorts=5
  update_Ki : Subsystem  Commented=on
  update_Kp : Subsystem  Commented=on
  w_n_des : Scope  Commented=on
  w_n_desired : Subsystem  Commented=on
  DesCurrent : Outport
  wires:
  Multiport Switch1/1 -> Gain10/1
  Rate Transition3/1 -> Gain9/1
  pos_exo/1 -> [pos_exo], Sin1/1
  vel_actuator/1 -> Subsystem3/1(x), [vel_act]
  [control_type] -> Multiport Switch1/1
  Sin1/1 -> Gain7/1
  control_type/1 -> [control_type]
  Product/1 -> actuation_terms/3, Sum10/1, actuation_terms1/3, Sum1/3  "hum_acc_ff"
  Subsystem3/1(dot_x) -> Gain6/1
  Constant/1 -> Product/2
  Gain9/1 -> Product/1
  Constant4/1 -> Filtering2/4(dt)
  Constant5/1 -> Filtering2/2(cutoff_freq [Hz])
  Constant3/1 -> Filtering2/3(reset_filter)
  vel_exo/1 -> [vel_exo], Scope/1, Filtering2/1(new)
  vel_hum/1 -> [vel_hum], Filtering1/1(new)
  Constant1/1 -> Filtering1/3(reset_filter)
  Constant6/1 -> Filtering1/2(cutoff_freq [Hz])
  Constant2/1 -> Filtering1/4(dt)
  Sqrt/1 -> w_n_des/1
  From9/1 -> w_n_desired/1(KneePosition)
  Constant7/1 -> Mux1/3
  update_Kp/1(Kp_acc) -> update_Ki/1(Kp_acc), Scope1/1, Mux1/1
  w_n_desired/1(w_n_sq) -> update_Kp/1(w_n_sq), Sqrt/1
  update_Ki/1(Ki_acc) -> Mux1/2, Scope1/2
  Mux1/1 -> Switch/1
  Subsystem1/1(dot_x) -> Rate Transition3/1
  Gain6/1 -> Sum1/2
  Gain10/1 -> DesCurrent/1  "DesCurrent"
  Sum7/1 -> Multiport Switch1/2
  pos_act/1 -> [pos_act]
  [pos_act] -> Sum4/1
  [pos_exo] -> Sum4/2
  Sum4/1 -> Gain/1
  Sum1/1 -> actuation_terms/2, Sum7/2  "act_inertia"
  Sum6/1 -> EposVelocityController/1
  Filtering2/1(filtered) -> Scope/2
  [vel_hum] -> Subsystem1/1(x)
  [vel_hum] -> Sum2/1
  [vel_exo] -> Sum2/2
  [vel_act] -> Sum9/2, Sum6/3
  [vel_hum] -> Rate Transition4/1
  Rate Transition4/1 -> actuation_terms1/5, Sum9/1, Sum6/1  "vel_hum"
  Gain/1 -> Sum5/3, actuation_terms1/2  "sea_torque"
  Sum3/1 -> Sum5/2
  Sum5/1 -> A_without_damping/1, A(z)/1(In1)
  int_torque_est/1 -> Sum8/2
  Sum8/1 -> PID Controller/1
  Constant8/1 -> Sum8/1  "ref"
  PID Controller/1 -> Gain1/1
  Manual Switch/1 -> actuation_terms/4, Sum7/1  "feedback"
  Sum2/1 -> Vel_PID_ideal_1ms/1, Vel_PID_nonideal_1ms/1, Vel_PID_nonideal_8ms/1
  A(z)/1(Out1) -> actuation_terms1/4, AzRef_X_VelErr/1, Sum6/2  "vel_adm_des"
  Sum9/1 -> AzRef_X_VelErr/2
  Vel_PID_nonideal_8ms/1 -> Rate Transition2/1
  Vel_PID_ideal_1ms/1 -> Manual Switch/1
  Gain7/1 -> Gain2/1  "exo_weight"
  Rate Transition2/1 -> Manual Switch1/1
  Manual Switch1/1 -> Manual Switch/2
  Vel_PID_nonideal_1ms/1 -> Manual Switch1/2
  Gain2/1 -> actuation_terms/1, Sum3/1, actuation_terms1/1, Sum1/1  "exo_weight"
  Sum10/1 -> Multiport Switch1/3
  EposVelocityController/1 -> Sum10/2

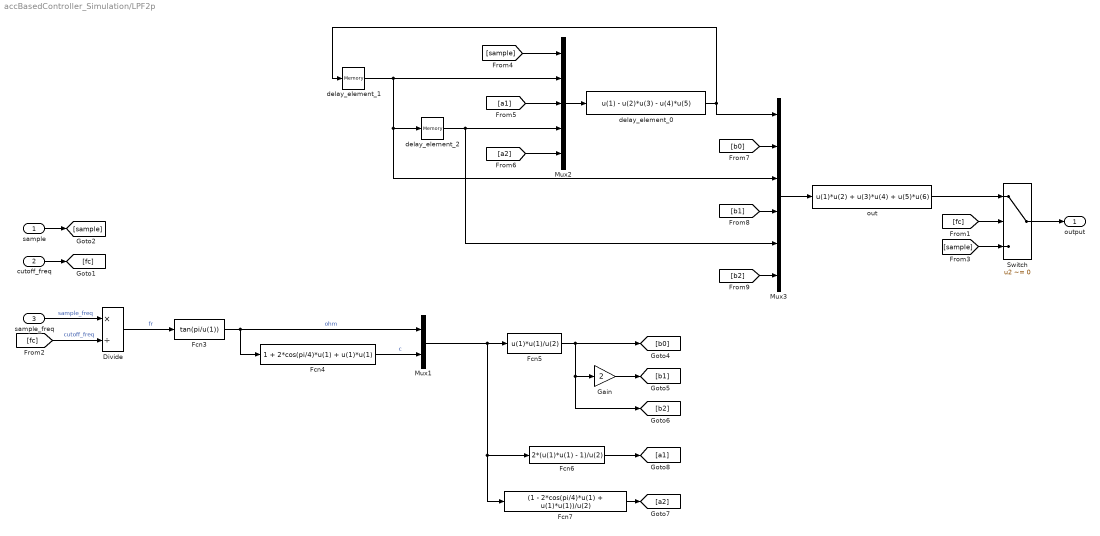
== system accBasedController_Simulation/LPF2p ==
  sample : Inport
  cutoff_freq : Inport  Port=2
  sample_freq : Inport  Port=3
  Divide : Product  Inputs=*/
  Fcn3 : Fcn  Expr=tan(pi/u(1))
  Fcn4 : Fcn  Expr=1 + 2*cos(pi/4)*u(1) + u(1)*u(1)
  Fcn5 : Fcn  Expr=u(1)*u(1)/u(2)
  Fcn6 : Fcn  Expr=2*(u(1)*u(1) - 1)/u(2)
  Fcn7 : Fcn  Expr=(1 - 2*cos(pi/4)*u(1) + u(1)*u(1))/u(2)
  Gain : Gain  Gain=2
  Mux1 : Mux  Inputs=2
  Mux2 : Mux  Inputs=5
  Mux3 : Mux  Inputs=6
  Switch : Switch  Criteria=u2 ~= 0
  delay_element_0 : Fcn  Expr=u(1) - u(2)*u(3) - u(4)*u(5)
  delay_element_1 : Memory  InheritSampleTime=on
  delay_element_2 : Memory  InheritSampleTime=on
  out : Fcn  Expr=u(1)*u(2) + u(3)*u(4) + u(5)*u(6)
  output : Outport
  wires:
  Switch/1 -> output/1
  cutoff_freq/1 -> [fc]
  [fc] -> Switch/2
  sample_freq/1 -> Divide/1  "sample_freq"
  [fc] -> Divide/2  "cutoff_freq"
  Divide/1 -> Fcn3/1  "fr"
  Mux1/1 -> Fcn7/1, Fcn6/1, Fcn5/1
  Fcn3/1 -> Mux1/1, Fcn4/1  "ohm"
  Fcn4/1 -> Mux1/2  "c"
  Fcn5/1 -> [b0], [b2], Gain/1
  Gain/1 -> [b1]
  Fcn6/1 -> [a1]
  Fcn7/1 -> [a2]
  sample/1 -> [sample]
  [sample] -> Switch/3
  delay_element_1/1 -> delay_element_2/1, Mux3/3, Mux2/2
  [sample] -> Mux2/1
  Mux2/1 -> delay_element_0/1
  [a1] -> Mux2/3
  delay_element_2/1 -> Mux2/4, Mux3/5
  [a2] -> Mux2/5
  out/1 -> Switch/1
  delay_element_0/1 -> delay_element_1/1, Mux3/1
  [b0] -> Mux3/2
  [b1] -> Mux3/4
  [b2] -> Mux3/6
  Mux3/1 -> out/1

== system accBasedController_Simulation/MeanAbsError ==
  ref : Inport
  state : Inport  Port=2
  Abs4 : Abs
  Mean1 : dspstat3/Mean  run=on  InputProcessing=Columns as channels (frame based)  reset_popup=None  directionMode=Each column  dimension=1  roiEnable=off  roiType=Rectangles  roiPortion=Entire ROI  roiOutput=Individual statistics for each ROI  roiFlag=off  roundingMode=Floor  overflowMode=off  outputDataTypeStr=Inherit: Same as accumulator  outputMin=[]  outputMax=[]  outputLastDataTypeStr=Inherit: Same as accumulator
  Sum2 : Sum  Inputs=|+-
  Error : Outport
  wires:
  state/1 -> Sum2/2
  Abs4/1 -> Mean1/1
  Sum2/1 -> Abs4/1
  Mean1/1 -> Error/1
  ref/1 -> Sum2/1

== system accBasedController_Simulation/MeanAbsError1 ==
  ref : Inport
  state : Inport  Port=2
  Abs4 : Abs
  Mean1 : dspstat3/Mean  run=on  InputProcessing=Columns as channels (frame based)  reset_popup=None  directionMode=Each column  dimension=1  roiEnable=off  roiType=Rectangles  roiPortion=Entire ROI  roiOutput=Individual statistics for each ROI  roiFlag=off  roundingMode=Floor  overflowMode=off  outputDataTypeStr=Inherit: Same as accumulator  outputMin=[]  outputMax=[]  outputLastDataTypeStr=Inherit: Same as accumulator
  Sum2 : Sum  Inputs=|+-
  Error : Outport
  wires:
  ref/1 -> Sum2/1
  Mean1/1 -> Error/1
  Sum2/1 -> Abs4/1
  Abs4/1 -> Mean1/1
  state/1 -> Sum2/2

== system accBasedController_Simulation/Subsystem ==
  x : Inport
  Constant12 : Constant  Value=1/dt
  Constant13 : Constant  Value=7
  Gain17 : Gain  Gain=1/(dt)
  LowPassFilter2p : Subsystem
  Sum : Sum  Inputs=|+-
  Unit Delay1 : UnitDelay  SampleTime=-1  HasFrameUpgradeWarning=on
  dot_x : Outport
  wires:
  Unit Delay1/1 -> Sum/2
  Sum/1 -> Gain17/1
  Gain17/1 -> LowPassFilter2p/1(sample)
  LowPassFilter2p/1(output) -> dot_x/1
  Constant12/1 -> LowPassFilter2p/3(sample_freq)
  x/1 -> Unit Delay1/1, Sum/1
  Constant13/1 -> LowPassFilter2p/2(cutoff_freq)

== system accBasedController_Simulation/Subsystem1 ==
  x : Inport
  Constant12 : Constant  Value=1/dt
  Constant13 : Constant  Value=7
  Gain17 : Gain  Gain=1/(dt)
  LowPassFilter2p : Subsystem
  Sum : Sum  Inputs=|+-
  Unit Delay1 : UnitDelay  SampleTime=-1  HasFrameUpgradeWarning=on
  dot_x : Outport
  wires:
  Constant13/1 -> LowPassFilter2p/2(cutoff_freq)
  x/1 -> Sum/1, Unit Delay1/1
  Constant12/1 -> LowPassFilter2p/3(sample_freq)
  LowPassFilter2p/1(output) -> dot_x/1
  Gain17/1 -> LowPassFilter2p/1(sample)
  Sum/1 -> Gain17/1
  Unit Delay1/1 -> Sum/2

== system accBasedController_Simulation/Subsystem2 ==
  x : Inport
  Constant12 : Constant  Value=1/dt
  Constant13 : Constant  Value=5
  Gain17 : Gain  Gain=1/(dt)
  LowPassFilter2p : Subsystem
  Sum : Sum  Inputs=|+-
  Unit Delay1 : UnitDelay  SampleTime=-1  HasFrameUpgradeWarning=on
  dot_x : Outport
  wires:
  Constant13/1 -> LowPassFilter2p/2(cutoff_freq)
  x/1 -> Sum/1, Unit Delay1/1
  Constant12/1 -> LowPassFilter2p/3(sample_freq)
  LowPassFilter2p/1(output) -> dot_x/1
  Gain17/1 -> LowPassFilter2p/1(sample)
  Sum/1 -> Gain17/1
  Unit Delay1/1 -> Sum/2

== system accBasedController_Simulation/Subsystem3 ==
  x : Inport
  Constant12 : Constant  Value=1/dt
  Constant13 : Constant  Value=10
  Gain17 : Gain  Gain=1/(dt)
  LowPassFilter2p : Subsystem
  Sum : Sum  Inputs=|+-
  Unit Delay1 : UnitDelay  SampleTime=-1  HasFrameUpgradeWarning=on
  dot_x : Outport
  wires:
  Constant13/1 -> LowPassFilter2p/2(cutoff_freq)
  x/1 -> Sum/1, Unit Delay1/1
  Constant12/1 -> LowPassFilter2p/3(sample_freq)
  LowPassFilter2p/1(output) -> dot_x/1
  Gain17/1 -> LowPassFilter2p/1(sample)
  Sum/1 -> Gain17/1
  Unit Delay1/1 -> Sum/2

== system accBasedController_Simulation/UnitDelay ==
  In1 : Inport
  Unit Delay : UnitDelay  SampleTime=-1  HasFrameUpgradeWarning=on
  y : Outport  VectorParamsAs1DForOutWhenUnconnected=off
  wires:
  Unit Delay/1 -> y/1
  In1/1 -> Unit Delay/1

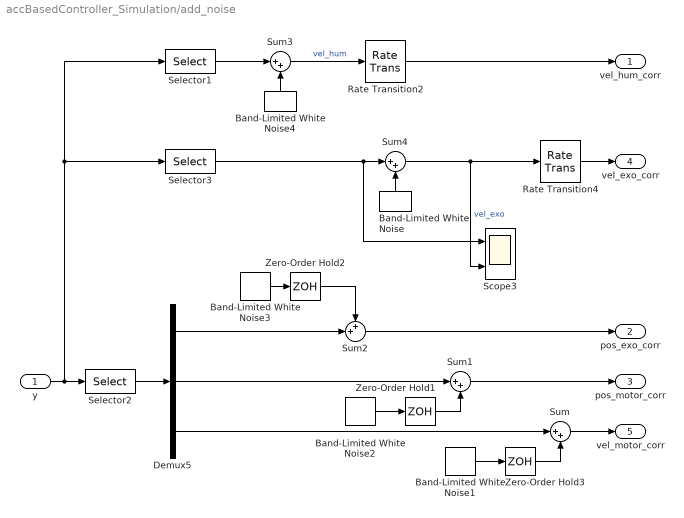
== system accBasedController_Simulation/add_noise ==
  y : Inport
  Band-Limited White Noise : simulink/Sources/Band-Limited White Noise  Cov=5.476e-6  Ts=dt  seed=[23341]  VectorParams1D=off
  Band-Limited White Noise1 : simulink/Sources/Band-Limited White Noise  Cov=1.096e-2  Ts=dt  seed=[23541]  VectorParams1D=off
  Band-Limited White Noise2 : simulink/Sources/Band-Limited White Noise  Cov=2.353e-6  Ts=dt  seed=[23543]  VectorParams1D=off
  Band-Limited White Noise3 : simulink/Sources/Band-Limited White Noise  Cov=9.412e-6  Ts=dt  seed=[87541]  VectorParams1D=off
  Band-Limited White Noise4 : simulink/Sources/Band-Limited White Noise  Cov=5.476e-6  Ts=dt  seed=[41236]  VectorParams1D=off
  Demux5 : Demux  Outputs=3
  Rate Transition2 : RateTransition  OutPortSampleTime=0.008
  Rate Transition4 : RateTransition  OutPortSampleTime=0.008
  Scope3 : Scope  NumInputPorts=2
  Selector1 : Selector  InputPortWidth=sensor_dim  IndexOptions=Index vector (dialog)  Indices=[v_h_idx]  OutputSizes=1
  Selector2 : Selector  InputPortWidth=sensor_dim  IndexOptions=Index vector (dialog)  Indices=[p_e_idx, p_m_idx, v_m_idx]  OutputSizes=1
  Selector3 : Selector  InputPortWidth=sensor_dim  IndexOptions=Index vector (dialog)  Indices=[v_e_idx]  OutputSizes=1
  Sum{,1,3..4} (4 alike) : Sum  Inputs=|++
  Sum2 : Sum  Inputs=++|
  Zero-Order Hold1 : ZeroOrderHold  SampleTime=dt
  Zero-Order Hold2 : ZeroOrderHold  SampleTime=dt
  Zero-Order Hold3 : ZeroOrderHold  SampleTime=dt
  vel_hum_corr : Outport
  pos_exo_corr : Outport  Port=2
  pos_motor_corr : Outport  Port=3
  vel_exo_corr : Outport  Port=4
  vel_motor_corr : Outport  Port=5
  wires:
  Selector2/1 -> Demux5/1
  Sum/1 -> vel_motor_corr/1
  Demux5/3 -> Sum/1
  Zero-Order Hold3/1 -> Sum/2
  y/1 -> Selector3/1, Selector1/1, Selector2/1
  Band-Limited White Noise1/1 -> Zero-Order Hold3/1
  Band-Limited White Noise2/1 -> Zero-Order Hold1/1
  Zero-Order Hold1/1 -> Sum1/2
  Sum1/1 -> pos_motor_corr/1
  Demux5/2 -> Sum1/1
  Band-Limited White Noise3/1 -> Zero-Order Hold2/1
  Sum2/1 -> pos_exo_corr/1
  Demux5/1 -> Sum2/2
  Zero-Order Hold2/1 -> Sum2/1
  Band-Limited White Noise4/1 -> Sum3/2
  Selector1/1 -> Sum3/1
  Sum3/1 -> Rate Transition2/1  "vel_hum"
  Rate Transition2/1 -> vel_hum_corr/1
  Selector3/1 -> Sum4/1, Scope3/1
  Sum4/1 -> Rate Transition4/1, Scope3/2  "vel_exo"
  Band-Limited White Noise/1 -> Sum4/2
  Rate Transition4/1 -> vel_exo_corr/1

== system accBasedController_Simulation/noise_resample_filtering ==
  vel_hum : Inport
  vel_exo : Inport  Port=2
  Band-Limited White Noise : simulink/Sources/Band-Limited White Noise  Cov=[dt*dt*0.3]  Ts=dt  seed=[23341]  VectorParams1D=off
  Band-Limited White Noise1 : simulink/Sources/Band-Limited White Noise  Cov=[dt*dt*0.3]  Ts=dt  seed=[41236]  VectorParams1D=off
  LowPassFilter2p : Subsystem
  LowPassFilter2p1 : Subsystem
  Rate Transition2 : RateTransition  OutPortSampleTime=0.008
  Rate Transition4 : RateTransition  OutPortSampleTime=0.008
  Scope3 : Scope  NumInputPorts=3
  Sum1 : Sum  Inputs=|++
  Sum2 : Sum  Inputs=|++
  XSENS_FC : Constant  Value=60
  XSENS_FC1 : Constant  Value=60
  XSENS_RATE : Constant  Value=120
  XSENS_RATE1 : Constant  Value=120
  ve_hum_filt : Outport
  vel_exo_filt : Outport  Port=2
  wires:
  vel_hum/1 -> Sum2/1
  XSENS_FC/1 -> LowPassFilter2p/2(cutoff_freq)
  LowPassFilter2p/1(output) -> ve_hum_filt/1  "vel_hum"
  XSENS_FC1/1 -> LowPassFilter2p1/2(cutoff_freq)
  Rate Transition4/1 -> LowPassFilter2p1/1(sample)
  vel_exo/1 -> Scope3/1, Sum1/1
  LowPassFilter2p1/1(output) -> vel_exo_filt/1, Scope3/3
  Sum2/1 -> Rate Transition2/1  "vel_hum"
  Sum1/1 -> Scope3/2, Rate Transition4/1  "vel_exo"
  Band-Limited White Noise1/1 -> Sum2/2
  Rate Transition2/1 -> LowPassFilter2p/1(sample)
  XSENS_RATE/1 -> LowPassFilter2p/3(sample_freq)
  Band-Limited White Noise/1 -> Sum1/2
  XSENS_RATE1/1 -> LowPassFilter2p1/3(sample_freq)

== system accBasedController_Simulation/update_Ki ==
  Kp_acc : Inport
  zeta : Inport  Port=2
  Bias : Bias  Bias=Je
  Gain2 : Gain  Gain=Ka
  Gain3 : Gain  Gain=2
  Product : Product
  Sqrt1 : Sqrt  SaturateOnIntegerOverflow=on
  Ki_acc : Outport
  wires:
  Bias/1 -> Gain2/1
  Gain2/1 -> Sqrt1/1
  Gain3/1 -> Ki_acc/1
  Kp_acc/1 -> Bias/1
  Sqrt1/1 -> Product/1
  Product/1 -> Gain3/1
  zeta/1 -> Product/2

== system accBasedController_Simulation/update_Kp ==
  w_n : Inport
  Constant : Constant  Value=Ka
  Divide : Product  Inputs=*/
  Gain1 : Gain  Gain=Je
  Square : Math  Operator=square  SaturateOnIntegerOverflow=on
  Sum : Sum  Inputs=|+-
  Kp_acc : Outport
  wires:
  Divide/1 -> Kp_acc/1
  Sum/1 -> Divide/1
  w_n/1 -> Square/1
  Constant/1 -> Sum/1
  Gain1/1 -> Sum/2
  Square/1 -> Divide/2, Gain1/1

== system accBasedController_Simulation/AccBasedController/A(z) ==
  In1 : Inport
  A(s) : TransferFcn  Numerator=[k_bar 0]  Denominator=[damping_d stiffness_d]
  Rate Transition1 : RateTransition  OutPortSampleTime=0.001
  Zero-Order Hold : ZeroOrderHold  SampleTime=-1
  Out1 : Outport
  wires:
  Zero-Order Hold/1 -> A(s)/1
  A(s)/1 -> Rate Transition1/1
  In1/1 -> Zero-Order Hold/1
  Rate Transition1/1 -> Out1/1

== system accBasedController_Simulation/AccBasedController/Filtering1 ==
  note: // get_filt_alpha - calculate a filter alpha
      | float AC_PID::get_filt_alpha(float filt_hz) const
      | {
      |     if (is_zero(filt_hz)) {
      |         return 1.0f;
      |     }
      |
      |     // calculate alpha
      |     float rc = 1 / (M_2PI * filt_hz);
      |     return _dt / (_dt + rc);
      | }
  note: e.g.:
      |
      | _target += get_filt_T_alpha() * (target - _target);
  new : Inport
  cutoff_freq [Hz] : Inport  Port=2
  reset_filter : Inport  Port=3
  dt : Inport  Port=4
  Constant6 : Constant
  Memory4 : Memory  InheritSampleTime=on
  Mux : Mux  Inputs=2
  Product5 : Product
  Subtract6 : Sum  Inputs=+-
  Subtract7 : Sum
  Switch : Switch  Criteria=u2 ~= 0
  Switch1 : Switch  Criteria=u2 ~= 0
  alpha : Fcn  Expr=u(1)/(u(1)+1/(2*pi*u(2)))
  filtered : Outport
  wires:
  Subtract7/1 -> Switch1/3
  Switch1/1 -> Memory4/1, filtered/1
  reset_filter/1 -> Switch1/2
  [alpha] -> Product5/1
  Switch/1 -> [alpha]
  Constant6/1 -> Switch/3
  new/1 -> Subtract6/1, Switch1/1
  Memory4/1 -> Subtract6/2, Subtract7/2
  Subtract6/1 -> Product5/2
  Product5/1 -> Subtract7/1
  Mux/1 -> alpha/1
  cutoff_freq [Hz]/1 -> Switch/2, Mux/2
  alpha/1 -> Switch/1
  dt/1 -> Mux/1
